simulink model "double_pend"  (R2019b)
settings: Solver=VariableStepAuto  StartTime=0.0  StopTime=10.0  RelTol=1e-3
values from neighbouring files (symbols this model uses):
  Bd = 50    [anujay_single_pendulum_same.m]    (also in connect_pend_runner.m; double_pend_setup.m = [50,0;0,50])
  dampener = 100    [anujay_single_pendulum_same.m]    (also in connect_pend.m; connect_pend_runner.m; double_pend_setup.m = [50, 0; 0, 50])
  Dm1 = 30    [anujay_single_pendulum_same.m]    (also in connect_pend.m; connect_pend_runner.m; double_pend_setup.m = [30,0;0,30])
  Kd = 50    [anujay_single_pendulum_same.m]    (also in connect_pend_runner.m; double_pend_setup.m = [50,0;0,50]; single_pend_runner.m = 500)
  Ked = 50    [anujay_single_pendulum_same.m]    (also in double_pend_setup.m = [ 100, 0; 0, 100])
  Kem = 50    [anujay_single_pendulum_same.m]    (also in double_pend_setup.m = [100, 0; 0, 100])
  Km1 = 30    [anujay_single_pendulum_same.m]    (also in connect_pend.m; connect_pend_runner.m; double_pend_setup.m = [30, 0; 0 30])
  l = [ 1.0, 1.5]    [double_pend_setup.m]
  l1 = 1.0    (= 1)    [connect_pend.m]    (also in connect_pend_runner.m; run.m)
  l2 = l1    (= 1)    [connect_pend_runner.m]    (also in single_pend_runner.m = 3)
  lambda2 = 1.2    [anujay_single_pendulum_same.m]    (also in connect_pend_runner.m = 3; double_pend_setup.m = [1.5, 0; 0 1.5])
  Md = 10    [anujay_single_pendulum_same.m]    (also in connect_pend_runner.m; double_pend_setup.m = [10, 0; 0, 10])
  me = 2.11  + mh    (= 13.934)    [anujay_single_pendulum_same.m]    (also in double_pend_setup.m = [ 2, 1] + mh)
  mh = 11.824    [anujay_single_pendulum_same.m]    (also in double_pend_setup.m = [2, 1])
  rho2 = 100    [anujay_single_pendulum_same.m]    (also in connect_pend_runner.m = 15; double_pend_setup.m = [100, 0; 0, 100])
  sat = 10    [double_pend_setup.m]
  spring = 100    [anujay_single_pendulum_same.m]    (also in connect_pend.m; connect_pend_runner.m; double_pend_setup.m = [50, 0; 0, 50])
undefined symbols (not defined in the file or in its folder): me2
libraries: simulink x2, robotcorelib x1
settings Model: Creator=nathanielgoldfarb  LastModifiedBy=nathanielgoldfarb
settings SolverCC: ZeroCrossAlgorithm=Adaptive
settings DebuggingCC: IgnoredZcDiagnostic=none  UnderSpecifiedDimensionMsg=warning

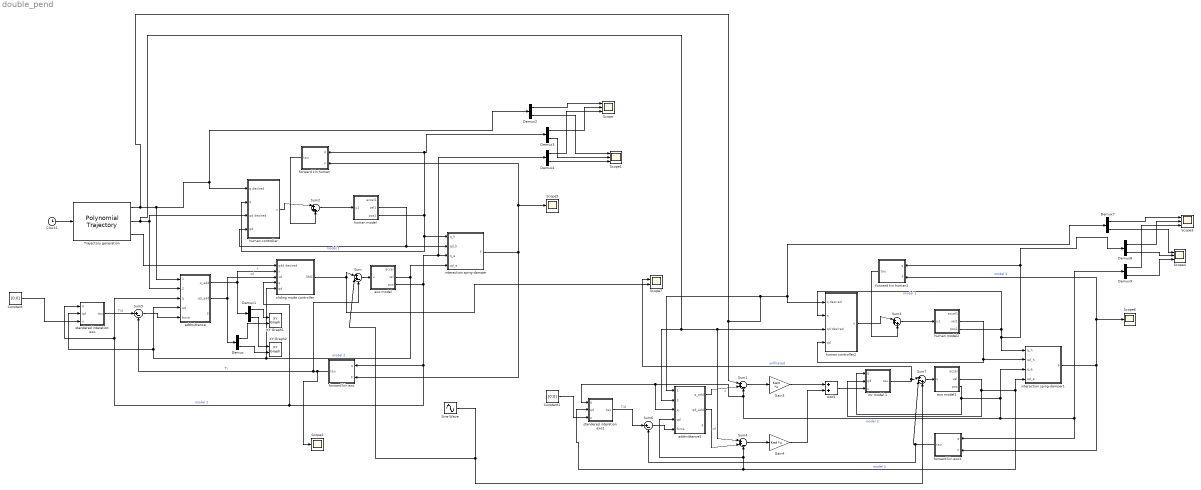
== system double_pend ==
  " interaction sping-damper" : Subsystem
  " interaction sping-damper1" : Subsystem
  Add1 : Sum
  Clock1 : Clock
  Constant : Constant  Value=[0;0]
  Constant1 : Constant  Value=[0;0]
  Demux{,1..4,7..9} (8 alike) : Demux  Outputs=2
  Gain3 : Gain  Gain=Kem  Multiplication=Matrix(K*u)
  Gain4 : Gain  Gain=Ked  Multiplication=Matrix(K*u)
  Scope{,1,3..4} (4 alike) : Scope  NumInputPorts=3
  Scope2 : Scope
  Scope5 : Scope
  Scope6 : Scope
  Scope7 : Scope  NumInputPorts=2
  Sine Wave : Sin  Amplitude=0  Frequency=4  SampleTime=0
  Sum : Sum  Inputs=|++-
  Sum1 : Sum  Inputs=|++-
  Sum2 : Sum  Inputs=|+++
  Sum3 : Sum  Inputs=|+++
  Sum4 : Sum  Inputs=|++-
  Sum5 : Sum  Inputs=|+-
  Sum6 : Sum  Inputs=|+-
  Sum7 : Sum  Inputs=|+-+
  Trajectory generation : robotcorelib/Polynomial Trajectory  WaypointSource=Internal  Waypoints="[ 0 , -pi;  0 -0.5*pi ]"  TimePoints=[ 0, 3]  TimeInterval=[ 1, 4 ]  Method=Cubic Polynomial  ParameterSource=Internal  VelocityBoundaryCondition=zeros( 2, 2 )  AccelerationBoundaryCondition=zeros( 2, 5 )  SimulateUsing=Interpreted execution
      settings: SourceProductName=Robotics System Toolbox  SourceProductBaseCode=RO
  XY Graph1 : simulink/Sinks/XY Graph  xmin=-5  xmax=5  ymin=-3  ymax=3  st=-1
  XY Graph2 : simulink/Sinks/XY Graph  xmin=-3  xmax=0.5  ymin=-2  ymax=2.2  st=-1
  addmittance : Subsystem
  addmittance1 : Subsystem
  exo model : Subsystem
  exo model1 : Subsystem
  forward kin exo : Subsystem
  forward kin exo1 : Subsystem
  forward kin human : Subsystem
  forward kin human1 : Subsystem
  human controller : Subsystem
  human controller2 : Subsystem
  human model : Subsystem
  human model2 : Subsystem
  inv model 1 : Subsystem
  sliding mode controller : Subsystem
  standered interation exo : Subsystem
  standered interation exo1 : Subsystem
  wires:
  addmittance/1(q_add) -> Demux1/1, sliding mode controller/2(x)  "x"
  Clock1/1 -> Trajectory generation/1
  Trajectory generation/3 -> sliding mode controller/1(qdd desired)
  human model/3(pos1) -> human controller/2(q), " interaction sping-damper"/1(q_h), Demux3/1, forward kin human/1(q)  "model 1"
  human model/2(vel1) -> human controller/4(qd), " interaction sping-damper"/2(qd_h)
  forward kin human/1(tau) -> Sum2/3
  " interaction sping-damper"/1(F) -> forward kin exo/2(F), forward kin human/2(F), Scope5/1
  exo model/2(vel) -> " interaction sping-damper"/4("qd_e "), standered interation exo/2(qd), addmittance/4(qd), sliding mode controller/5(qd)  "model 2"
  Sum5/1 -> addmittance/5(force)
  exo model/3(pos) -> Demux4/1, " interaction sping-damper"/3(q_e), sliding mode controller/4(q), standered interation exo/1(q), addmittance/3(q), forward kin exo/1(q)  "model 2"
  addmittance/2(qd_add) -> Demux/1, sliding mode controller/3(xd)  "xd"
  standered interation exo/1("tau ") -> Sum5/1  "Tid"
  Constant/1 -> standered interation exo/3("u ")
  Demux/2 -> XY Graph2/2
  Demux/1 -> XY Graph1/2
  Demux1/1 -> XY Graph1/1
  Demux1/2 -> XY Graph2/1
  forward kin exo/1(tau) -> Scope2/1, Sum5/2, Sum/3  "Ti"
  Demux2/1 -> Scope/1
  Demux3/1 -> Scope/2
  Demux4/1 -> Scope/3
  Demux2/2 -> Scope1/1
  Demux3/2 -> Scope1/2
  Demux4/2 -> Scope1/3
  exo model1/2(vel) -> inv model 1/2(qd), " interaction sping-damper1"/4("qd_e "), Sum4/3, addmittance1/4(qd), standered interation exo1/2(qd)  "model 2"
  Demux7/2 -> Scope4/1
  Demux9/1 -> Scope3/3
  forward kin human1/1(tau) -> Sum3/3
  Demux7/1 -> Scope3/1
  Demux8/2 -> Scope4/2
  exo model1/3(pos) -> inv model 1/1(q), " interaction sping-damper1"/3(q_e), Sum1/3, addmittance1/3(q), standered interation exo1/1(q), Demux9/1, forward kin exo1/1(q)  "model 2"
  Demux9/2 -> Scope4/3
  human model2/3(pos1) -> " interaction sping-damper1"/1(q_h), forward kin human1/1(q), Demux8/1, human controller2/2(q)  "model 1"
  Demux8/1 -> Scope3/2
  human model2/2(vel1) -> human controller2/4(qd), " interaction sping-damper1"/2(qd_h)
  Trajectory generation/1 -> Demux7/1, human controller2/1(q desired), addmittance1/1(q desird), Sum1/1, addmittance/1(q desird), human controller/1(q desired), Demux2/1
  " interaction sping-damper1"/1(F) -> forward kin exo1/2(F), forward kin human1/2(F), Scope6/1  "model 2"
  Sum4/1 -> Gain4/1
  Gain4/1 -> Add1/2
  Trajectory generation/2 -> addmittance1/2(qd desird), Sum4/1, human controller2/3(qd desired), human controller/3(qd desired), addmittance/2(qd desird)
  Gain3/1 -> Add1/1
  Sum1/1 -> Gain3/1
  Sine Wave/1 -> Sum7/3, Sum/2
  human controller/1(u) -> Sum2/1
  Sum2/1 -> human model/1(u1)
  human controller2/1(u) -> Sum3/1
  Sum3/1 -> human model2/1(u1)
  Add1/1 -> inv model 1/3("u ")
  inv model 1/1("tau ") -> Sum7/1, Scope7/1  "unfiltered"
  Sum7/1 -> exo model1/1(u)
  forward kin exo1/1(tau) -> Sum6/2, Sum7/2
  Sum/1 -> exo model/1(u)
  sliding mode controller/1(SMC) -> Sum/1, Scope7/2
  Constant1/1 -> standered interation exo1/3("u ")
  standered interation exo1/1("tau ") -> Sum6/1  "Tid"
  addmittance1/1(q_add) -> Sum1/2  "x"
  addmittance1/2(qd_add) -> Sum4/2  "xd"
  Sum6/1 -> addmittance1/5(force)

== system double_pend/ interaction sping-damper ==
  q_h : Inport
  qd_h : Inport  Port=2
  q_e : Inport  Port=3
  "qd_e " : Inport  Port=4
  Mux : Mux  Inputs=2
  Subsystem : Subsystem
  Subsystem1 : Subsystem
  forward kin : Subsystem
  forward kin2 : Subsystem
  F : Outport
  wires:
  qd_h/1 -> forward kin/2(qd)
  q_h/1 -> forward kin/1("q ")
  "qd_e "/1 -> forward kin2/2(qd)
  q_e/1 -> forward kin2/1("q ")
  forward kin/1(pos1) -> Subsystem/1(x human)
  forward kin/3(vel1) -> Subsystem/2("xd human ")
  forward kin2/1(pos1) -> Subsystem/3(x exo)
  forward kin2/3(vel1) -> Subsystem/4(xd exo)
  forward kin/2(pos2) -> Subsystem1/1(x human)
  forward kin2/2(pos2) -> Subsystem1/3(x exo)
  forward kin/4(vel2) -> Subsystem1/2("xd human ")
  forward kin2/4(vel2) -> Subsystem1/4(xd exo)
  Subsystem/1(F) -> Mux/1
  Subsystem1/1(F) -> Mux/2
  Mux/1 -> F/1

== system double_pend/ interaction sping-damper1 ==
  q_h : Inport
  qd_h : Inport  Port=2
  q_e : Inport  Port=3
  "qd_e " : Inport  Port=4
  Mux : Mux  Inputs=2
  Subsystem : Subsystem
  Subsystem1 : Subsystem
  forward kin : Subsystem
  forward kin2 : Subsystem
  F : Outport
  wires:
  qd_h/1 -> forward kin/2(qd)
  q_h/1 -> forward kin/1("q ")
  "qd_e "/1 -> forward kin2/2(qd)
  q_e/1 -> forward kin2/1("q ")
  forward kin/1(pos1) -> Subsystem/1(x human)
  forward kin/3(vel1) -> Subsystem/2("xd human ")
  forward kin2/1(pos1) -> Subsystem/3(x exo)
  forward kin2/3(vel1) -> Subsystem/4(xd exo)
  forward kin/2(pos2) -> Subsystem1/1(x human)
  forward kin2/2(pos2) -> Subsystem1/3(x exo)
  forward kin/4(vel2) -> Subsystem1/2("xd human ")
  forward kin2/4(vel2) -> Subsystem1/4(xd exo)
  Subsystem/1(F) -> Mux/1
  Subsystem1/1(F) -> Mux/2
  Mux/1 -> F/1

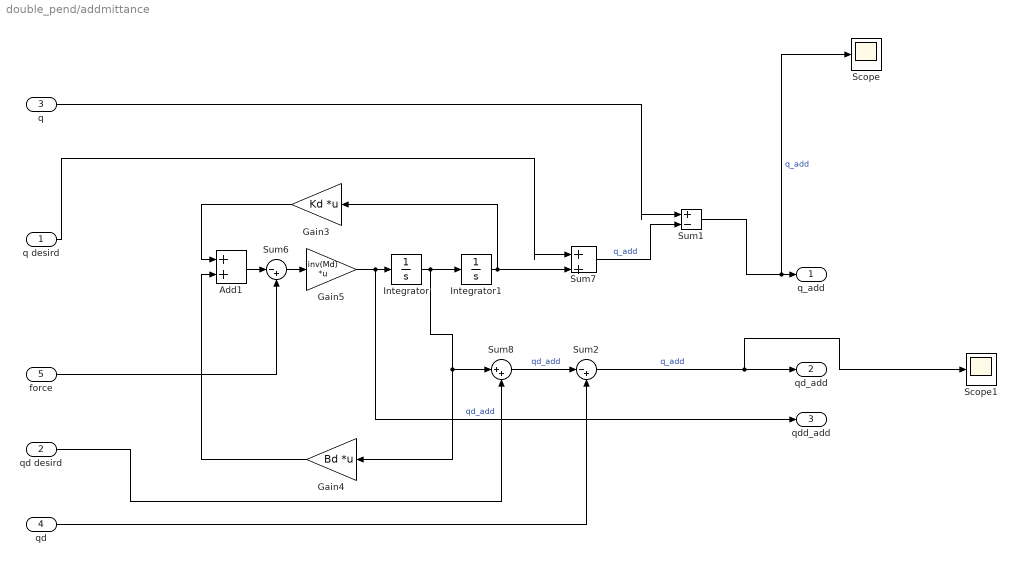
== system double_pend/addmittance ==
  q desird : Inport
  qd desird : Inport  Port=2
  q : Inport  Port=3
  qd : Inport  Port=4
  force : Inport  Port=5
  Add1 : Sum
  Gain3 : Gain  Gain=Kd  Multiplication=Matrix(K*u)
  Gain4 : Gain  Gain=Bd  Multiplication=Matrix(K*u)
  Gain5 : Gain  Gain=inv(Md)  Multiplication=Matrix(K*u)
  Integrator : Integrator
  Integrator1 : Integrator  InitialCondition=[-pi, 0.5*pi]
  Scope : Scope
  Scope1 : Scope
  Sum1 : Sum  Inputs=|+-
  Sum2 : Sum  Inputs=|-+
  Sum6 : Sum  Inputs=|-+
  Sum7 : Sum  Inputs=|++
  Sum8 : Sum  Inputs=|++
  q_add : Outport
  qd_add : Outport  Port=2
  qdd_add : Outport  Port=3
  wires:
  Add1/1 -> Sum6/1
  force/1 -> Sum6/2
  qd desird/1 -> Sum8/2
  Gain5/1 -> qdd_add/1, Integrator/1  "qd_add"
  Sum6/1 -> Gain5/1
  Gain4/1 -> Add1/2
  Gain3/1 -> Add1/1
  Integrator/1 -> Gain4/1, Sum8/1, Integrator1/1
  q desird/1 -> Sum7/1
  Integrator1/1 -> Sum7/2, Gain3/1
  qd/1 -> Sum2/2
  Sum2/1 -> Scope1/1, qd_add/1  "q_add"
  Sum7/1 -> Sum1/2  "q_add"
  q/1 -> Sum1/1
  Sum1/1 -> Scope/1, q_add/1  "q_add"
  Sum8/1 -> Sum2/1  "qd_add"

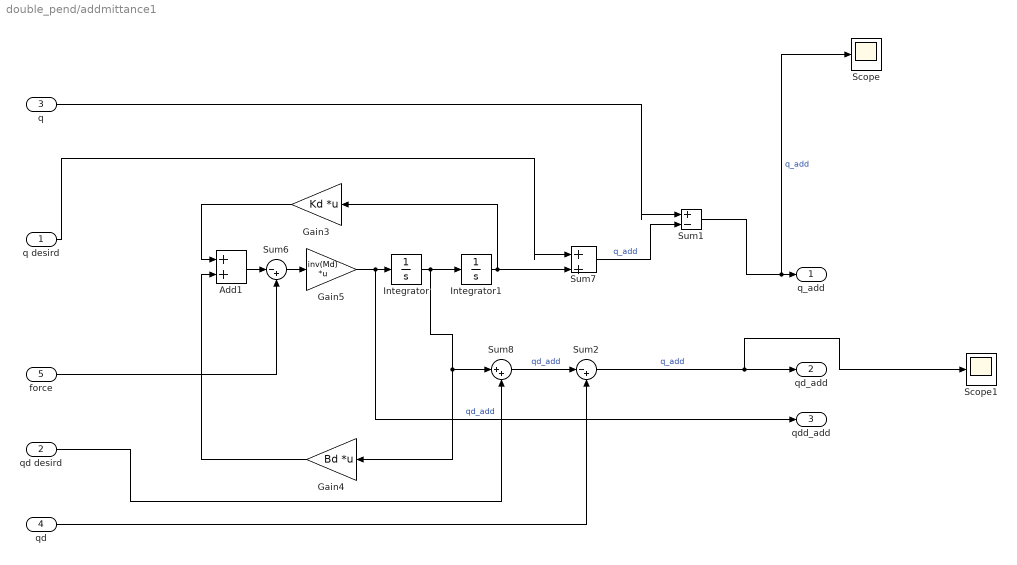
== system double_pend/addmittance1 ==
  q desird : Inport
  qd desird : Inport  Port=2
  q : Inport  Port=3
  qd : Inport  Port=4
  force : Inport  Port=5
  Add1 : Sum
  Gain3 : Gain  Gain=Kd  Multiplication=Matrix(K*u)
  Gain4 : Gain  Gain=Bd  Multiplication=Matrix(K*u)
  Gain5 : Gain  Gain=inv(Md)  Multiplication=Matrix(K*u)
  Integrator : Integrator
  Integrator1 : Integrator  InitialCondition=[-pi, 0.5*pi]
  Scope : Scope
  Scope1 : Scope
  Sum1 : Sum  Inputs=|+-
  Sum2 : Sum  Inputs=|-+
  Sum6 : Sum  Inputs=|-+
  Sum7 : Sum  Inputs=|++
  Sum8 : Sum  Inputs=|++
  q_add : Outport
  qd_add : Outport  Port=2
  qdd_add : Outport  Port=3
  wires:
  Add1/1 -> Sum6/1
  force/1 -> Sum6/2
  qd desird/1 -> Sum8/2
  Gain5/1 -> qdd_add/1, Integrator/1  "qd_add"
  Sum6/1 -> Gain5/1
  Gain4/1 -> Add1/2
  Gain3/1 -> Add1/1
  Integrator/1 -> Gain4/1, Sum8/1, Integrator1/1
  q desird/1 -> Sum7/1
  Integrator1/1 -> Sum7/2, Gain3/1
  qd/1 -> Sum2/2
  Sum2/1 -> Scope1/1, qd_add/1  "q_add"
  Sum7/1 -> Sum1/2  "q_add"
  q/1 -> Sum1/1
  Sum1/1 -> Scope/1, q_add/1  "q_add"
  Sum8/1 -> Sum2/1  "qd_add"

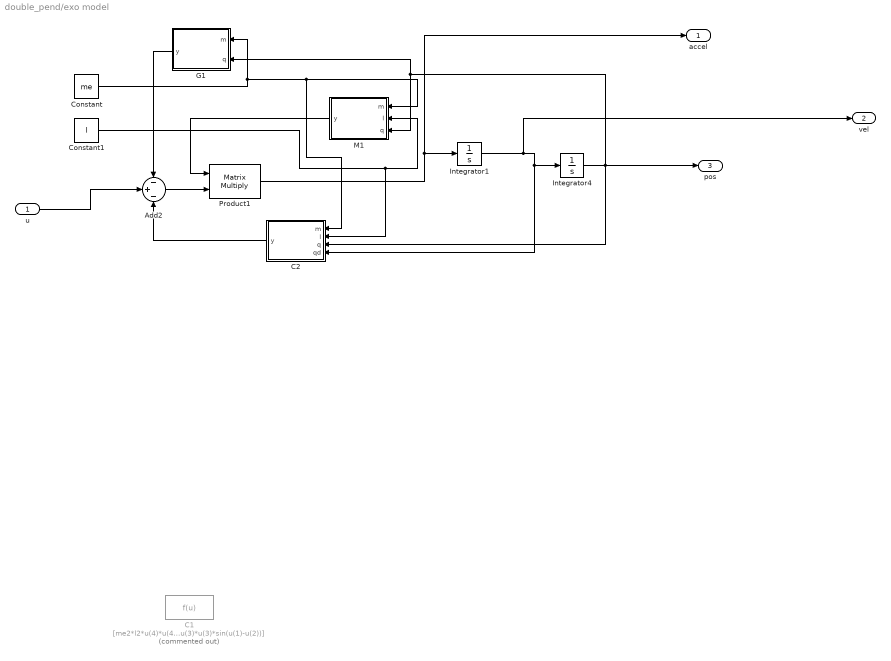
== system double_pend/exo model ==
  u : Inport
  Add2 : Sum  Inputs=-+-
  C1 : Fcn  Commented=on  Expr=[me2*l2*u(4)*u(4)*sin(u(1)-u(2)); -me2*l1*u(3)*u(3)*sin(u(1)-u(2))]
  C2 : MATLAB Function  TreatAsAtomicUnit=on
  Constant : Constant  Value=me
  Constant1 : Constant  Value=l
  G1 : MATLAB Function  TreatAsAtomicUnit=on
  Integrator1 : Integrator  InitialCondition=[0;0]
  Integrator4 : Integrator  InitialCondition=[0.01;0.01]
  M1 : MATLAB Function  TreatAsAtomicUnit=on
  Product1 : Product  Multiplication=Matrix(*)
  accel : Outport
  vel : Outport  Port=2
  pos : Outport  Port=3
  wires:
  Constant/1 -> C2/1(m), M1/1(m), G1/1(m)
  M1/1(y) -> Product1/1
  Add2/1 -> Product1/2
  C2/1(y) -> Add2/3
  G1/1(y) -> Add2/1
  u/1 -> Add2/2
  Product1/1 -> accel/1, Integrator1/1
  Constant1/1 -> C2/2(l), M1/2(l)
  Integrator4/1 -> pos/1, G1/2(q), M1/3(q), C2/3(q)
  Integrator1/1 -> vel/1, C2/4(qd), Integrator4/1

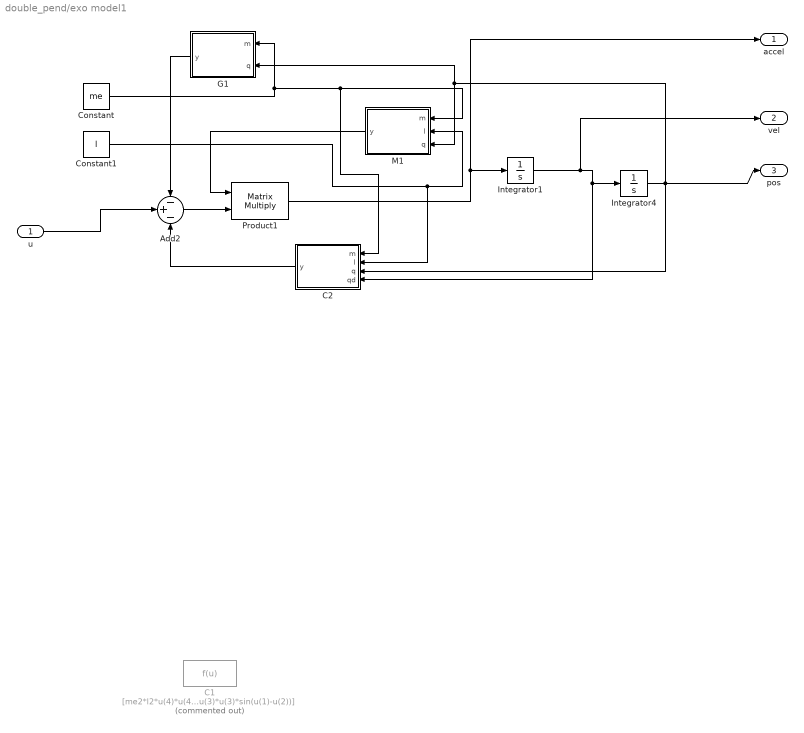
== system double_pend/exo model1 ==
  u : Inport
  Add2 : Sum  Inputs=-+-
  C1 : Fcn  Commented=on  Expr=[me2*l2*u(4)*u(4)*sin(u(1)-u(2)); -me2*l1*u(3)*u(3)*sin(u(1)-u(2))]
  C2 : MATLAB Function  TreatAsAtomicUnit=on
  Constant : Constant  Value=me
  Constant1 : Constant  Value=l
  G1 : MATLAB Function  TreatAsAtomicUnit=on
  Integrator1 : Integrator  InitialCondition=[0;0]
  Integrator4 : Integrator  InitialCondition=[0.01;0.01]
  M1 : MATLAB Function  TreatAsAtomicUnit=on
  Product1 : Product  Multiplication=Matrix(*)
  accel : Outport
  vel : Outport  Port=2
  pos : Outport  Port=3
  wires:
  Constant/1 -> C2/1(m), M1/1(m), G1/1(m)
  M1/1(y) -> Product1/1
  Add2/1 -> Product1/2
  C2/1(y) -> Add2/3
  G1/1(y) -> Add2/1
  u/1 -> Add2/2
  Product1/1 -> accel/1, Integrator1/1
  Constant1/1 -> C2/2(l), M1/2(l)
  Integrator1/1 -> vel/1, C2/4(qd), Integrator4/1
  Integrator4/1 -> pos/1, G1/2(q), M1/3(q), C2/3(q)

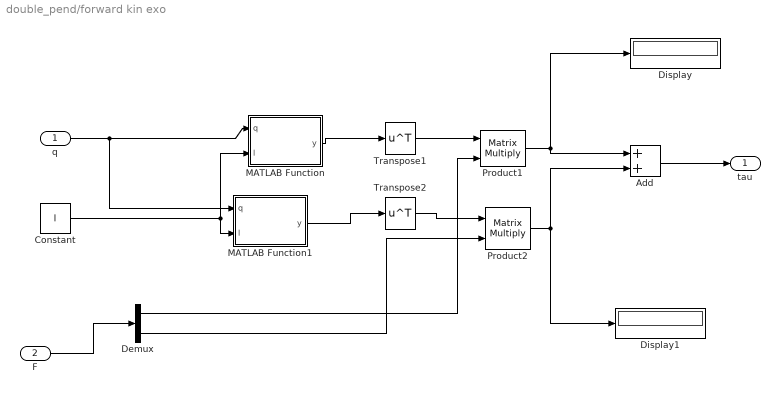
== system double_pend/forward kin exo ==
  q : Inport
  F : Inport  Port=2
  Add : Sum
  Constant : Constant  Value=l
  Demux : Demux  Outputs=2
  Display : Display
  Display1 : Display
  MATLAB Function : MATLAB Function  TreatAsAtomicUnit=on
  MATLAB Function1 : MATLAB Function  TreatAsAtomicUnit=on
  Product1 : Product  Multiplication=Matrix(*)
  Product2 : Product  Multiplication=Matrix(*)
  Transpose1 : Math  Operator=transpose  SignedPower=off  SaturateOnIntegerOverflow=on
  Transpose2 : Math  Operator=transpose  SignedPower=off  SaturateOnIntegerOverflow=on
  tau : Outport
  wires:
  Product1/1 -> Add/1, Display/1
  F/1 -> Demux/1
  q/1 -> MATLAB Function1/1(q), MATLAB Function/1(q)
  Constant/1 -> MATLAB Function/2(l), MATLAB Function1/2(l)
  Add/1 -> tau/1
  Demux/2 -> Product2/2
  Transpose2/1 -> Product2/1
  Demux/1 -> Product1/2
  Product2/1 -> Add/2, Display1/1
  MATLAB Function1/1(y) -> Transpose2/1
  MATLAB Function/1(y) -> Transpose1/1
  Transpose1/1 -> Product1/1

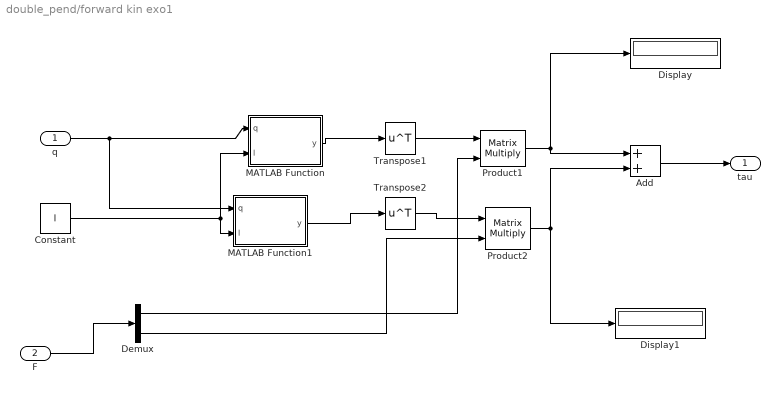
== system double_pend/forward kin exo1 ==
  q : Inport
  F : Inport  Port=2
  Add : Sum
  Constant : Constant  Value=l
  Demux : Demux  Outputs=2
  Display : Display
  Display1 : Display
  MATLAB Function : MATLAB Function  TreatAsAtomicUnit=on
  MATLAB Function1 : MATLAB Function  TreatAsAtomicUnit=on
  Product1 : Product  Multiplication=Matrix(*)
  Product2 : Product  Multiplication=Matrix(*)
  Transpose1 : Math  Operator=transpose  SignedPower=off  SaturateOnIntegerOverflow=on
  Transpose2 : Math  Operator=transpose  SignedPower=off  SaturateOnIntegerOverflow=on
  tau : Outport
  wires:
  Product1/1 -> Add/1, Display/1
  F/1 -> Demux/1
  q/1 -> MATLAB Function1/1(q), MATLAB Function/1(q)
  Constant/1 -> MATLAB Function/2(l), MATLAB Function1/2(l)
  Add/1 -> tau/1
  Demux/2 -> Product2/2
  Transpose2/1 -> Product2/1
  Demux/1 -> Product1/2
  Product2/1 -> Add/2, Display1/1
  MATLAB Function1/1(y) -> Transpose2/1
  MATLAB Function/1(y) -> Transpose1/1
  Transpose1/1 -> Product1/1

== system double_pend/forward kin human ==
  q : Inport
  F : Inport  Port=2
  Add : Sum
  Constant : Constant  Value=l
  Demux : Demux  Outputs=2
  Display : Display
  Display1 : Display
  MATLAB Function : MATLAB Function  TreatAsAtomicUnit=on
  MATLAB Function1 : MATLAB Function  TreatAsAtomicUnit=on
  Product1 : Product  Multiplication=Matrix(*)
  Product2 : Product  Multiplication=Matrix(*)
  Transpose1 : Math  Operator=transpose  SignedPower=off  SaturateOnIntegerOverflow=on
  Transpose2 : Math  Operator=transpose  SignedPower=off  SaturateOnIntegerOverflow=on
  tau : Outport
  wires:
  q/1 -> MATLAB Function1/1(q), MATLAB Function/1(q)
  Demux/2 -> Product2/2
  F/1 -> Demux/1
  Demux/1 -> Product1/2
  Transpose1/1 -> Product1/1
  Transpose2/1 -> Product2/1
  MATLAB Function1/1(y) -> Transpose2/1
  MATLAB Function/1(y) -> Transpose1/1
  Constant/1 -> MATLAB Function/2(l), MATLAB Function1/2(l)
  Add/1 -> tau/1
  Product1/1 -> Add/1, Display/1
  Product2/1 -> Add/2, Display1/1

== system double_pend/forward kin human1 ==
  q : Inport
  F : Inport  Port=2
  Add : Sum
  Constant : Constant  Value=l
  Demux : Demux  Outputs=2
  Display : Display
  Display1 : Display
  MATLAB Function : MATLAB Function  TreatAsAtomicUnit=on
  MATLAB Function1 : MATLAB Function  TreatAsAtomicUnit=on
  Product1 : Product  Multiplication=Matrix(*)
  Product2 : Product  Multiplication=Matrix(*)
  Transpose1 : Math  Operator=transpose  SignedPower=off  SaturateOnIntegerOverflow=on
  Transpose2 : Math  Operator=transpose  SignedPower=off  SaturateOnIntegerOverflow=on
  tau : Outport
  wires:
  q/1 -> MATLAB Function1/1(q), MATLAB Function/1(q)
  Demux/2 -> Product2/2
  F/1 -> Demux/1
  Demux/1 -> Product1/2
  Transpose1/1 -> Product1/1
  Transpose2/1 -> Product2/1
  MATLAB Function1/1(y) -> Transpose2/1
  MATLAB Function/1(y) -> Transpose1/1
  Constant/1 -> MATLAB Function/2(l), MATLAB Function1/2(l)
  Add/1 -> tau/1
  Product1/1 -> Add/1, Display/1
  Product2/1 -> Add/2, Display1/1

== system double_pend/human controller ==
  q desired : Inport
  q : Inport  Port=2
  qd desired : Inport  Port=3
  qd : Inport  Port=4
  Add2 : Sum
  Gain1 : Gain  Gain=Km1  Multiplication=Matrix(K*u)
  Gain2 : Gain  Gain=Dm1  Multiplication=Matrix(K*u)
  Saturation : Saturate  UpperLimit=sat  LowerLimit=-sat
  Scope2 : Scope  NumInputPorts=3
  Sum1 : Sum  Inputs=|+-
  Sum3 : Sum  Inputs=|-+
  inv model 1 : Subsystem
  u : Outport
  wires:
  Sum1/1 -> Gain2/1
  qd/1 -> inv model 1/2(qd), Sum1/2
  Sum3/1 -> Gain1/1
  Gain2/1 -> Add2/2
  q desired/1 -> Sum3/2
  Add2/1 -> inv model 1/3("u ")
  Gain1/1 -> Add2/1
  inv model 1/1("tau ") -> Scope2/1, Saturation/1  "unfiltered"
  qd desired/1 -> Sum1/1
  q/1 -> Sum3/1, inv model 1/1(q)
  Saturation/1 -> u/1, Scope2/3, Scope2/2  "filtered"

== system double_pend/human controller2 ==
  q desired : Inport
  q : Inport  Port=2
  qd desired : Inport  Port=3
  qd : Inport  Port=4
  Add2 : Sum
  Gain1 : Gain  Gain=Km1  Multiplication=Matrix(K*u)
  Gain2 : Gain  Gain=Dm1  Multiplication=Matrix(K*u)
  Saturation : Saturate  UpperLimit=sat  LowerLimit=-sat
  Scope2 : Scope  NumInputPorts=3
  Sum1 : Sum  Inputs=|+-
  Sum3 : Sum  Inputs=|-+
  inv model 1 : Subsystem
  u : Outport
  wires:
  Sum1/1 -> Gain2/1
  qd/1 -> inv model 1/2(qd), Sum1/2
  Sum3/1 -> Gain1/1
  Gain2/1 -> Add2/2
  q desired/1 -> Sum3/2
  Add2/1 -> inv model 1/3("u ")
  Gain1/1 -> Add2/1
  inv model 1/1("tau ") -> Scope2/1, Saturation/1  "unfiltered"
  qd desired/1 -> Sum1/1
  q/1 -> Sum3/1, inv model 1/1(q)
  Saturation/1 -> u/1, Scope2/3, Scope2/2  "filtered"

== system double_pend/human model ==
  u1 : Inport
  Add2 : Sum  Inputs=-+-
  C : MATLAB Function  TreatAsAtomicUnit=on
  Constant : Constant  Value=mh
  Constant1 : Constant  Value=l
  G : MATLAB Function  TreatAsAtomicUnit=on
  Integrator1 : Integrator  InitialCondition=[0;0]
  Integrator4 : Integrator  InitialCondition=[0.01;0.01]
  M : MATLAB Function  TreatAsAtomicUnit=on
  Product1 : Product  Multiplication=Matrix(*)
  accel1 : Outport
  vel1 : Outport  Port=2
  pos1 : Outport  Port=3
  wires:
  C/1(y) -> Add2/3
  M/1(y) -> Product1/1
  G/1(y) -> Add2/1
  Integrator4/1 -> C/3(q), pos1/1, G/2(q), M/3(q)
  u1/1 -> Add2/2
  Product1/1 -> accel1/1, Integrator1/1
  Integrator1/1 -> vel1/1, C/4(qd), Integrator4/1
  Add2/1 -> Product1/2
  Constant/1 -> C/1(m), M/1(m), G/1(m)
  Constant1/1 -> C/2(l), M/2(l)

== system double_pend/human model2 ==
  u1 : Inport
  Add2 : Sum  Inputs=-+-
  C : MATLAB Function  TreatAsAtomicUnit=on
  Constant : Constant  Value=mh
  Constant1 : Constant  Value=l
  G : MATLAB Function  TreatAsAtomicUnit=on
  Integrator1 : Integrator  InitialCondition=[0;0]
  Integrator4 : Integrator  InitialCondition=[0.01;0.01]
  M : MATLAB Function  TreatAsAtomicUnit=on
  Product1 : Product  Multiplication=Matrix(*)
  accel1 : Outport
  vel1 : Outport  Port=2
  pos1 : Outport  Port=3
  wires:
  C/1(y) -> Add2/3
  M/1(y) -> Product1/1
  G/1(y) -> Add2/1
  Integrator4/1 -> C/3(q), pos1/1, G/2(q), M/3(q)
  u1/1 -> Add2/2
  Product1/1 -> accel1/1, Integrator1/1
  Integrator1/1 -> vel1/1, C/4(qd), Integrator4/1
  Add2/1 -> Product1/2
  Constant/1 -> C/1(m), M/1(m), G/1(m)
  Constant1/1 -> C/2(l), M/2(l)

== system double_pend/inv model 1 ==
  q : Inport
  qd : Inport  Port=2
  "u " : Inport  Port=3
  Add2 : Sum  Inputs=+++
  C2 : MATLAB Function  TreatAsAtomicUnit=on
  Constant : Constant  Value=me
  Constant1 : Constant  Value=l
  G1 : MATLAB Function  TreatAsAtomicUnit=on
  M1 : MATLAB Function  TreatAsAtomicUnit=on
  Product : Product  Multiplication=Matrix(*)
  "tau " : Outport
  wires:
  G1/1(y) -> Add2/3
  C2/1(y) -> Add2/2
  q/1 -> G1/2(q), C2/3(q), M1/3(q)
  qd/1 -> C2/4(qd)
  M1/1(y) -> Product/1
  Product/1 -> Add2/1
  Constant/1 -> G1/1(m), C2/1(m), M1/1(m)
  Constant1/1 -> C2/2(l), M1/2(l)
  "u "/1 -> Product/2
  Add2/1 -> "tau "/1

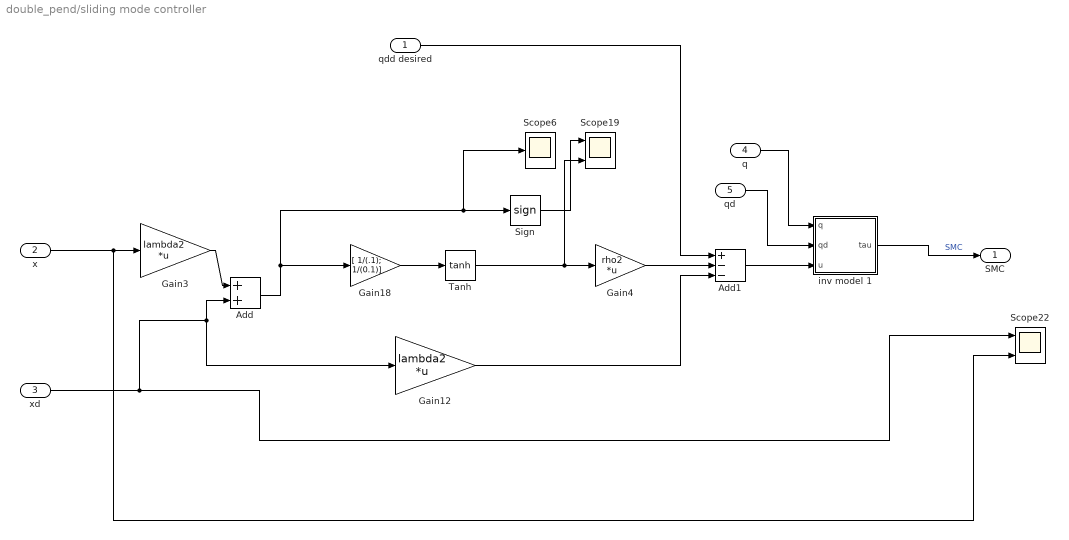
== system double_pend/sliding mode controller ==
  qdd desired : Inport
  x : Inport  Port=2
  xd : Inport  Port=3
  q : Inport  Port=4
  qd : Inport  Port=5
  Add : Sum
  Add1 : Sum  Inputs=+--
  Gain12 : Gain  Gain=lambda2  Multiplication=Matrix(K*u)
  Gain18 : Gain  Gain=[ 1/(.1); 1/(0.1)]
  Gain3 : Gain  Gain=lambda2  Multiplication=Matrix(K*u)
  Gain4 : Gain  Gain=rho2  Multiplication=Matrix(K*u)
  Scope19 : Scope  NumInputPorts=2
  Scope22 : Scope  NumInputPorts=2
  Scope6 : Scope
  Sign : Signum
  Tanh : Trigonometry  Operator=tanh
  inv model 1 : Subsystem
  SMC : Outport
  wires:
  Gain18/1 -> Tanh/1
  Gain12/1 -> Add1/3
  Gain3/1 -> Add/1
  inv model 1/1("tau ") -> SMC/1  "SMC"
  x/1 -> Scope22/2, Gain3/1
  xd/1 -> Add/2, Gain12/1, Scope22/1
  Add/1 -> Scope6/1, Sign/1, Gain18/1
  Add1/1 -> inv model 1/3("u ")
  Sign/1 -> Scope19/1
  Gain4/1 -> Add1/2
  qdd desired/1 -> Add1/1
  Tanh/1 -> Gain4/1, Scope19/2
  q/1 -> inv model 1/1(q)
  qd/1 -> inv model 1/2(qd)

== system double_pend/standered interation exo ==
  q : Inport
  qd : Inport  Port=2
  "u " : Inport  Port=3
  Add2 : Sum  Inputs=+++
  C2 : MATLAB Function  TreatAsAtomicUnit=on
  Constant : Constant  Value=me
  Constant1 : Constant  Value=l
  G1 : MATLAB Function  TreatAsAtomicUnit=on
  M : MATLAB Function  TreatAsAtomicUnit=on
  Product : Product  Multiplication=Matrix(*)
  "tau " : Outport
  wires:
  Add2/1 -> "tau "/1
  C2/1(y) -> Add2/2
  Product/1 -> Add2/1
  G1/1(y) -> Add2/3
  q/1 -> G1/2(q), C2/3(q), M/3(q)
  Constant/1 -> C2/1(m), M/1(m), G1/1(m)
  M/1(y) -> Product/1
  "u "/1 -> Product/2
  qd/1 -> C2/4(qd)
  Constant1/1 -> C2/2(l), M/2(l)

== system double_pend/standered interation exo1 ==
  q : Inport
  qd : Inport  Port=2
  "u " : Inport  Port=3
  Add2 : Sum  Inputs=+++
  C2 : MATLAB Function  TreatAsAtomicUnit=on
  Constant : Constant  Value=me
  Constant1 : Constant  Value=l
  G1 : MATLAB Function  TreatAsAtomicUnit=on
  M : MATLAB Function  TreatAsAtomicUnit=on
  Product : Product  Multiplication=Matrix(*)
  "tau " : Outport
  wires:
  Add2/1 -> "tau "/1
  C2/1(y) -> Add2/2
  Product/1 -> Add2/1
  G1/1(y) -> Add2/3
  q/1 -> G1/2(q), C2/3(q), M/3(q)
  Constant/1 -> C2/1(m), M/1(m), G1/1(m)
  M/1(y) -> Product/1
  "u "/1 -> Product/2
  qd/1 -> C2/4(qd)
  Constant1/1 -> C2/2(l), M/2(l)

== system double_pend/ interaction sping-damper/Subsystem ==
  x human : Inport
  "xd human " : Inport  Port=2
  x exo : Inport  Port=3
  xd exo : Inport  Port=4
  Gain3 : Gain  Gain=spring  Multiplication=Matrix(K*u)
  Gain4 : Gain  Gain=dampener  Multiplication=Matrix(K*u)
  Subtract : Sum  Inputs=-+
  Subtract1 : Sum  Inputs=-+
  Subtract2 : Sum
  F : Outport
  wires:
  Subtract2/1 -> F/1
  xd exo/1 -> Subtract1/2
  Gain4/1 -> Subtract2/2
  Subtract/1 -> Gain3/1
  Subtract1/1 -> Gain4/1
  x exo/1 -> Subtract/2
  x human/1 -> Subtract/1
  "xd human "/1 -> Subtract1/1
  Gain3/1 -> Subtract2/1

== system double_pend/ interaction sping-damper/Subsystem1 ==
  x human : Inport
  "xd human " : Inport  Port=2
  x exo : Inport  Port=3
  xd exo : Inport  Port=4
  Gain3 : Gain  Gain=spring  Multiplication=Matrix(K*u)
  Gain4 : Gain  Gain=dampener  Multiplication=Matrix(K*u)
  Subtract : Sum  Inputs=-+
  Subtract1 : Sum  Inputs=-+
  Subtract2 : Sum
  F : Outport
  wires:
  Subtract2/1 -> F/1
  xd exo/1 -> Subtract1/2
  Gain4/1 -> Subtract2/2
  Subtract/1 -> Gain3/1
  Subtract1/1 -> Gain4/1
  x exo/1 -> Subtract/2
  x human/1 -> Subtract/1
  "xd human "/1 -> Subtract1/1
  Gain3/1 -> Subtract2/1

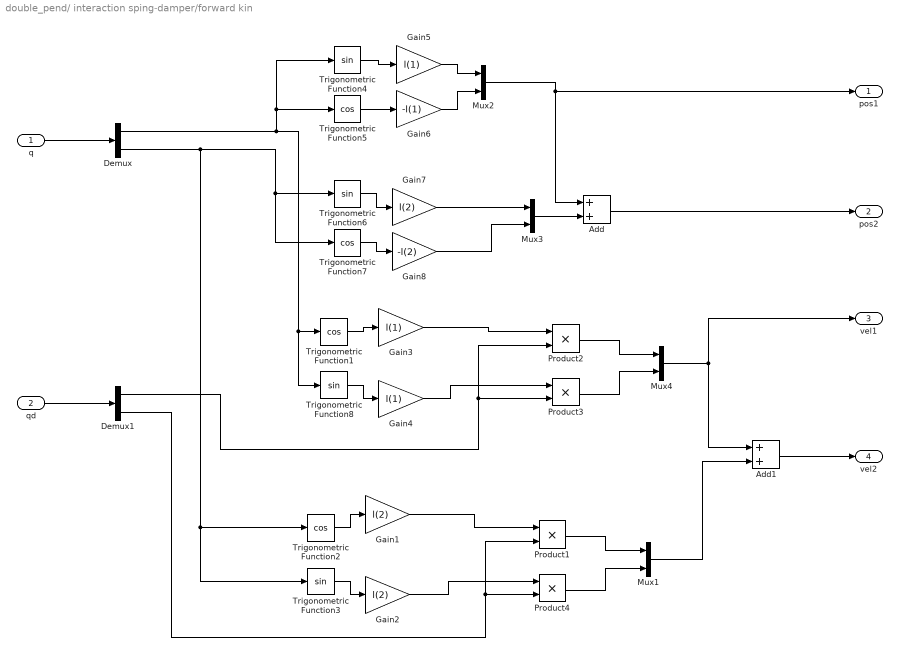
== system double_pend/ interaction sping-damper/forward kin ==
  "q " : Inport
  qd : Inport  Port=2
  Add : Sum
  Add1 : Sum
  Demux : Demux  Outputs=2
  Demux1 : Demux  Outputs=2
  Gain1 : Gain  Gain=l(2)
  Gain2 : Gain  Gain=l(2)
  Gain3 : Gain  Gain=l(1)
  Gain4 : Gain  Gain=l(1)
  Gain5 : Gain  Gain=l(1)
  Gain6 : Gain  Gain=-l(1)
  Gain7 : Gain  Gain=l(2)
  Gain8 : Gain  Gain=-l(2)
  Mux{1..4} (4 alike) : Mux  Inputs=2
  Product{1..4} (4 alike) : Product
  Trigonometric Function{1..2,5,7} (4 alike) : Trigonometry  Operator=cos
  Trigonometric Function{3..4,6,8} (4 alike) : Trigonometry
  pos1 : Outport
  pos2 : Outport  Port=2
  vel1 : Outport  Port=3
  vel2 : Outport  Port=4
  wires:
  "q "/1 -> Demux/1
  qd/1 -> Demux1/1
  Gain6/1 -> Mux2/2
  Trigonometric Function4/1 -> Gain5/1
  Gain5/1 -> Mux2/1
  Trigonometric Function5/1 -> Gain6/1
  Demux/1 -> Trigonometric Function8/1, Trigonometric Function1/1, Trigonometric Function5/1, Trigonometric Function4/1
  Trigonometric Function6/1 -> Gain7/1
  Gain8/1 -> Mux3/2
  Trigonometric Function7/1 -> Gain8/1
  Demux/2 -> Trigonometric Function3/1, Trigonometric Function2/1, Trigonometric Function7/1, Trigonometric Function6/1
  Gain7/1 -> Mux3/1
  Mux3/1 -> Add/2
  Trigonometric Function1/1 -> Gain3/1
  Gain3/1 -> Product2/1
  Demux1/1 -> Product3/2, Product2/2
  Trigonometric Function8/1 -> Gain4/1
  Gain4/1 -> Product3/1
  Product2/1 -> Mux4/1
  Product3/1 -> Mux4/2
  Trigonometric Function3/1 -> Gain2/1
  Trigonometric Function2/1 -> Gain1/1
  Product4/1 -> Mux1/2
  Demux1/2 -> Product4/2, Product1/2
  Gain2/1 -> Product4/1
  Product1/1 -> Mux1/1
  Gain1/1 -> Product1/1
  Mux4/1 -> Add1/1, vel1/1
  Mux1/1 -> Add1/2
  Add/1 -> pos2/1
  Mux2/1 -> Add/1, pos1/1
  Add1/1 -> vel2/1

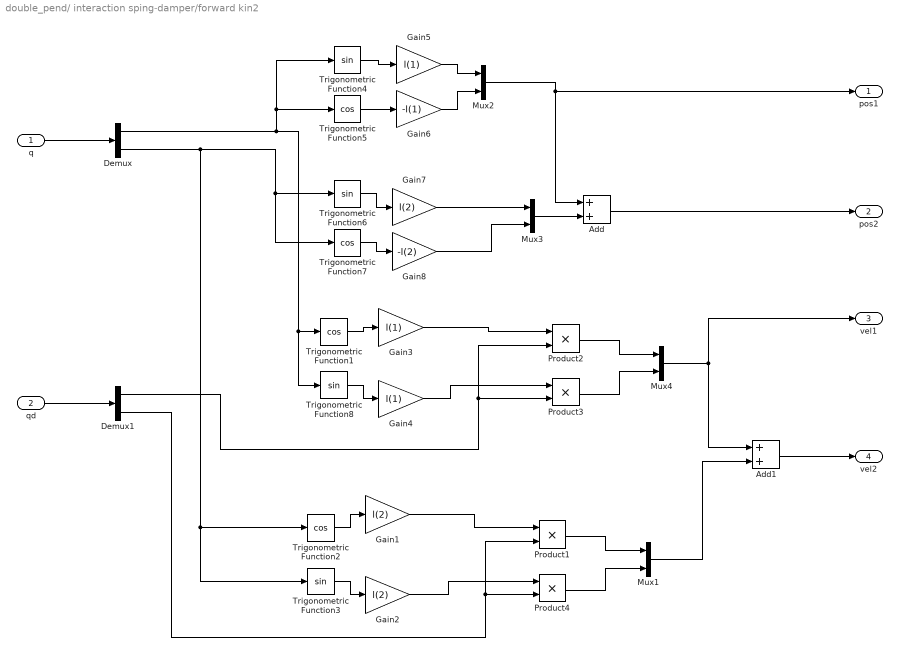
== system double_pend/ interaction sping-damper/forward kin2 ==
  "q " : Inport
  qd : Inport  Port=2
  Add : Sum
  Add1 : Sum
  Demux : Demux  Outputs=2
  Demux1 : Demux  Outputs=2
  Gain1 : Gain  Gain=l(2)
  Gain2 : Gain  Gain=l(2)
  Gain3 : Gain  Gain=l(1)
  Gain4 : Gain  Gain=l(1)
  Gain5 : Gain  Gain=l(1)
  Gain6 : Gain  Gain=-l(1)
  Gain7 : Gain  Gain=l(2)
  Gain8 : Gain  Gain=-l(2)
  Mux{1..4} (4 alike) : Mux  Inputs=2
  Product{1..4} (4 alike) : Product
  Trigonometric Function{1..2,5,7} (4 alike) : Trigonometry  Operator=cos
  Trigonometric Function{3..4,6,8} (4 alike) : Trigonometry
  pos1 : Outport
  pos2 : Outport  Port=2
  vel1 : Outport  Port=3
  vel2 : Outport  Port=4
  wires:
  "q "/1 -> Demux/1
  qd/1 -> Demux1/1
  Gain6/1 -> Mux2/2
  Trigonometric Function4/1 -> Gain5/1
  Gain5/1 -> Mux2/1
  Trigonometric Function5/1 -> Gain6/1
  Demux/1 -> Trigonometric Function8/1, Trigonometric Function1/1, Trigonometric Function5/1, Trigonometric Function4/1
  Trigonometric Function6/1 -> Gain7/1
  Gain8/1 -> Mux3/2
  Trigonometric Function7/1 -> Gain8/1
  Demux/2 -> Trigonometric Function3/1, Trigonometric Function2/1, Trigonometric Function7/1, Trigonometric Function6/1
  Gain7/1 -> Mux3/1
  Mux3/1 -> Add/2
  Trigonometric Function1/1 -> Gain3/1
  Gain3/1 -> Product2/1
  Demux1/1 -> Product3/2, Product2/2
  Trigonometric Function8/1 -> Gain4/1
  Gain4/1 -> Product3/1
  Product2/1 -> Mux4/1
  Product3/1 -> Mux4/2
  Trigonometric Function3/1 -> Gain2/1
  Trigonometric Function2/1 -> Gain1/1
  Product4/1 -> Mux1/2
  Demux1/2 -> Product4/2, Product1/2
  Gain2/1 -> Product4/1
  Product1/1 -> Mux1/1
  Gain1/1 -> Product1/1
  Mux4/1 -> Add1/1, vel1/1
  Mux1/1 -> Add1/2
  Add/1 -> pos2/1
  Mux2/1 -> Add/1, pos1/1
  Add1/1 -> vel2/1

== system double_pend/ interaction sping-damper1/Subsystem ==
  x human : Inport
  "xd human " : Inport  Port=2
  x exo : Inport  Port=3
  xd exo : Inport  Port=4
  Gain3 : Gain  Gain=spring  Multiplication=Matrix(K*u)
  Gain4 : Gain  Gain=dampener  Multiplication=Matrix(K*u)
  Subtract : Sum  Inputs=-+
  Subtract1 : Sum  Inputs=-+
  Subtract2 : Sum
  F : Outport
  wires:
  Subtract2/1 -> F/1
  xd exo/1 -> Subtract1/2
  Gain4/1 -> Subtract2/2
  Subtract/1 -> Gain3/1
  Subtract1/1 -> Gain4/1
  x exo/1 -> Subtract/2
  x human/1 -> Subtract/1
  "xd human "/1 -> Subtract1/1
  Gain3/1 -> Subtract2/1

== system double_pend/ interaction sping-damper1/Subsystem1 ==
  x human : Inport
  "xd human " : Inport  Port=2
  x exo : Inport  Port=3
  xd exo : Inport  Port=4
  Gain3 : Gain  Gain=spring  Multiplication=Matrix(K*u)
  Gain4 : Gain  Gain=dampener  Multiplication=Matrix(K*u)
  Subtract : Sum  Inputs=-+
  Subtract1 : Sum  Inputs=-+
  Subtract2 : Sum
  F : Outport
  wires:
  Subtract2/1 -> F/1
  xd exo/1 -> Subtract1/2
  Gain4/1 -> Subtract2/2
  Subtract/1 -> Gain3/1
  Subtract1/1 -> Gain4/1
  x exo/1 -> Subtract/2
  x human/1 -> Subtract/1
  "xd human "/1 -> Subtract1/1
  Gain3/1 -> Subtract2/1

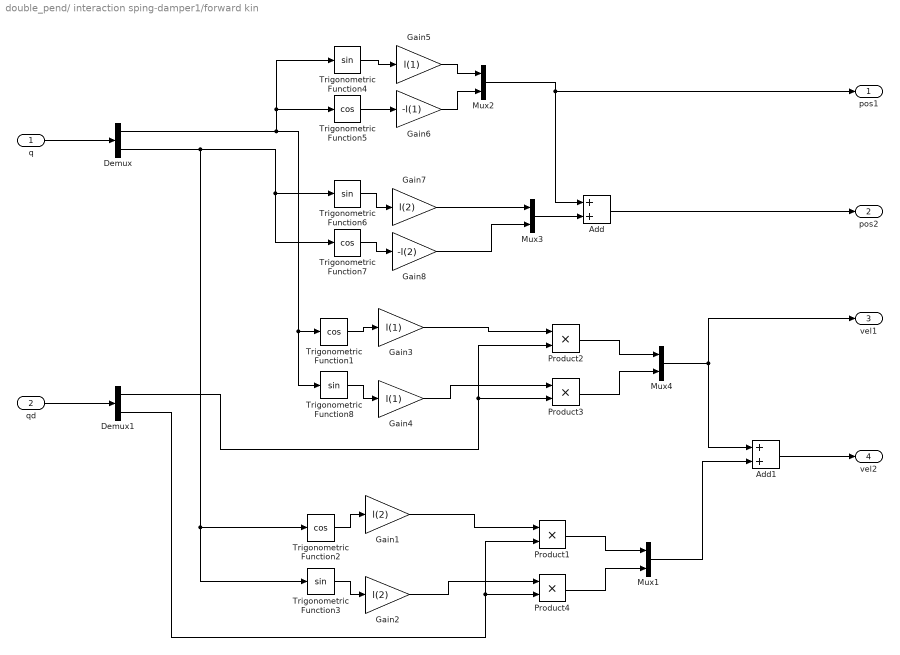
== system double_pend/ interaction sping-damper1/forward kin ==
  "q " : Inport
  qd : Inport  Port=2
  Add : Sum
  Add1 : Sum
  Demux : Demux  Outputs=2
  Demux1 : Demux  Outputs=2
  Gain1 : Gain  Gain=l(2)
  Gain2 : Gain  Gain=l(2)
  Gain3 : Gain  Gain=l(1)
  Gain4 : Gain  Gain=l(1)
  Gain5 : Gain  Gain=l(1)
  Gain6 : Gain  Gain=-l(1)
  Gain7 : Gain  Gain=l(2)
  Gain8 : Gain  Gain=-l(2)
  Mux{1..4} (4 alike) : Mux  Inputs=2
  Product{1..4} (4 alike) : Product
  Trigonometric Function{1..2,5,7} (4 alike) : Trigonometry  Operator=cos
  Trigonometric Function{3..4,6,8} (4 alike) : Trigonometry
  pos1 : Outport
  pos2 : Outport  Port=2
  vel1 : Outport  Port=3
  vel2 : Outport  Port=4
  wires:
  "q "/1 -> Demux/1
  qd/1 -> Demux1/1
  Gain6/1 -> Mux2/2
  Trigonometric Function4/1 -> Gain5/1
  Gain5/1 -> Mux2/1
  Trigonometric Function5/1 -> Gain6/1
  Demux/1 -> Trigonometric Function8/1, Trigonometric Function1/1, Trigonometric Function5/1, Trigonometric Function4/1
  Trigonometric Function6/1 -> Gain7/1
  Gain8/1 -> Mux3/2
  Trigonometric Function7/1 -> Gain8/1
  Demux/2 -> Trigonometric Function3/1, Trigonometric Function2/1, Trigonometric Function7/1, Trigonometric Function6/1
  Gain7/1 -> Mux3/1
  Mux3/1 -> Add/2
  Trigonometric Function1/1 -> Gain3/1
  Gain3/1 -> Product2/1
  Demux1/1 -> Product3/2, Product2/2
  Trigonometric Function8/1 -> Gain4/1
  Gain4/1 -> Product3/1
  Product2/1 -> Mux4/1
  Product3/1 -> Mux4/2
  Trigonometric Function3/1 -> Gain2/1
  Trigonometric Function2/1 -> Gain1/1
  Product4/1 -> Mux1/2
  Demux1/2 -> Product4/2, Product1/2
  Gain2/1 -> Product4/1
  Product1/1 -> Mux1/1
  Gain1/1 -> Product1/1
  Mux4/1 -> Add1/1, vel1/1
  Mux1/1 -> Add1/2
  Add/1 -> pos2/1
  Mux2/1 -> Add/1, pos1/1
  Add1/1 -> vel2/1

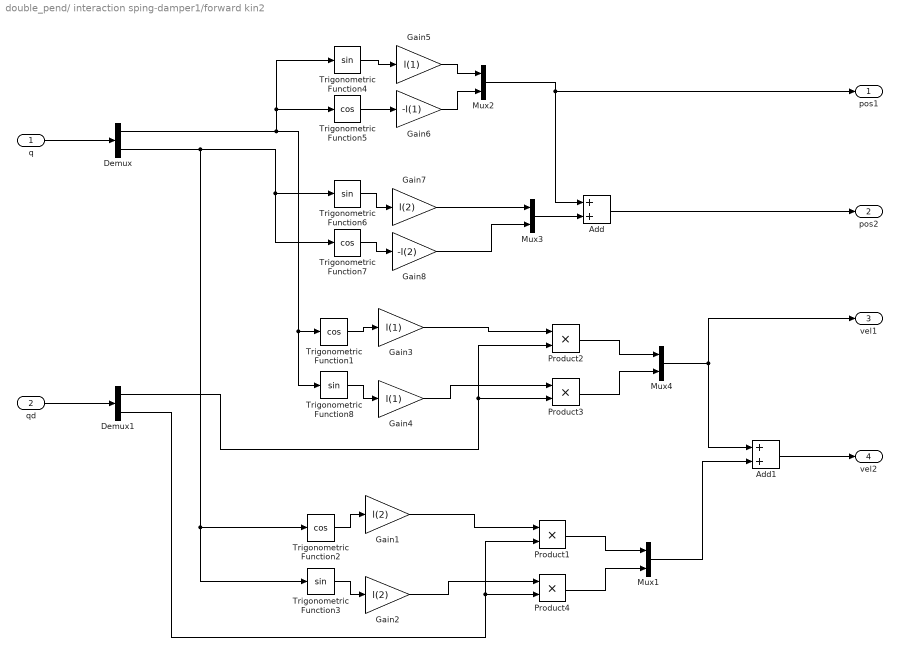
== system double_pend/ interaction sping-damper1/forward kin2 ==
  "q " : Inport
  qd : Inport  Port=2
  Add : Sum
  Add1 : Sum
  Demux : Demux  Outputs=2
  Demux1 : Demux  Outputs=2
  Gain1 : Gain  Gain=l(2)
  Gain2 : Gain  Gain=l(2)
  Gain3 : Gain  Gain=l(1)
  Gain4 : Gain  Gain=l(1)
  Gain5 : Gain  Gain=l(1)
  Gain6 : Gain  Gain=-l(1)
  Gain7 : Gain  Gain=l(2)
  Gain8 : Gain  Gain=-l(2)
  Mux{1..4} (4 alike) : Mux  Inputs=2
  Product{1..4} (4 alike) : Product
  Trigonometric Function{1..2,5,7} (4 alike) : Trigonometry  Operator=cos
  Trigonometric Function{3..4,6,8} (4 alike) : Trigonometry
  pos1 : Outport
  pos2 : Outport  Port=2
  vel1 : Outport  Port=3
  vel2 : Outport  Port=4
  wires:
  "q "/1 -> Demux/1
  qd/1 -> Demux1/1
  Gain6/1 -> Mux2/2
  Trigonometric Function4/1 -> Gain5/1
  Gain5/1 -> Mux2/1
  Trigonometric Function5/1 -> Gain6/1
  Demux/1 -> Trigonometric Function8/1, Trigonometric Function1/1, Trigonometric Function5/1, Trigonometric Function4/1
  Trigonometric Function6/1 -> Gain7/1
  Gain8/1 -> Mux3/2
  Trigonometric Function7/1 -> Gain8/1
  Demux/2 -> Trigonometric Function3/1, Trigonometric Function2/1, Trigonometric Function7/1, Trigonometric Function6/1
  Gain7/1 -> Mux3/1
  Mux3/1 -> Add/2
  Trigonometric Function1/1 -> Gain3/1
  Gain3/1 -> Product2/1
  Demux1/1 -> Product3/2, Product2/2
  Trigonometric Function8/1 -> Gain4/1
  Gain4/1 -> Product3/1
  Product2/1 -> Mux4/1
  Product3/1 -> Mux4/2
  Trigonometric Function3/1 -> Gain2/1
  Trigonometric Function2/1 -> Gain1/1
  Product4/1 -> Mux1/2
  Demux1/2 -> Product4/2, Product1/2
  Gain2/1 -> Product4/1
  Product1/1 -> Mux1/1
  Gain1/1 -> Product1/1
  Mux4/1 -> Add1/1, vel1/1
  Mux1/1 -> Add1/2
  Add/1 -> pos2/1
  Mux2/1 -> Add/1, pos1/1
  Add1/1 -> vel2/1

== system double_pend/human controller/inv model 1 ==
  q : Inport
  qd : Inport  Port=2
  "u " : Inport  Port=3
  Add2 : Sum  Inputs=+++
  C2 : MATLAB Function  TreatAsAtomicUnit=on
  Constant : Constant  Value=mh
  Constant1 : Constant  Value=l
  G1 : MATLAB Function  TreatAsAtomicUnit=on
  M1 : MATLAB Function  TreatAsAtomicUnit=on
  Product : Product  Multiplication=Matrix(*)
  "tau " : Outport
  wires:
  G1/1(y) -> Add2/3
  C2/1(y) -> Add2/2
  Add2/1 -> "tau "/1
  q/1 -> G1/2(q), C2/3(q), M1/3(q)
  qd/1 -> C2/4(qd)
  M1/1(y) -> Product/1
  Product/1 -> Add2/1
  "u "/1 -> Product/2
  Constant/1 -> G1/1(m), C2/1(m), M1/1(m)
  Constant1/1 -> C2/2(l), M1/2(l)

== system double_pend/human controller2/inv model 1 ==
  q : Inport
  qd : Inport  Port=2
  "u " : Inport  Port=3
  Add2 : Sum  Inputs=+++
  C2 : MATLAB Function  TreatAsAtomicUnit=on
  Constant : Constant  Value=mh
  Constant1 : Constant  Value=l
  G1 : MATLAB Function  TreatAsAtomicUnit=on
  M1 : MATLAB Function  TreatAsAtomicUnit=on
  Product : Product  Multiplication=Matrix(*)
  "tau " : Outport
  wires:
  G1/1(y) -> Add2/3
  C2/1(y) -> Add2/2
  Add2/1 -> "tau "/1
  q/1 -> G1/2(q), C2/3(q), M1/3(q)
  qd/1 -> C2/4(qd)
  M1/1(y) -> Product/1
  Product/1 -> Add2/1
  "u "/1 -> Product/2
  Constant/1 -> G1/1(m), C2/1(m), M1/1(m)
  Constant1/1 -> C2/2(l), M1/2(l)

== system double_pend/sliding mode controller/inv model 1 ==
  q : Inport
  qd : Inport  Port=2
  "u " : Inport  Port=3
  Add2 : Sum  Inputs=+++
  C2 : MATLAB Function  TreatAsAtomicUnit=on
  Constant : Constant  Value=me
  Constant1 : Constant  Value=l
  G1 : MATLAB Function  TreatAsAtomicUnit=on
  M1 : MATLAB Function  TreatAsAtomicUnit=on
  Product : Product  Multiplication=Matrix(*)
  "tau " : Outport
  wires:
  G1/1(y) -> Add2/3
  C2/1(y) -> Add2/2
  Add2/1 -> "tau "/1
  q/1 -> G1/2(q), C2/3(q), M1/3(q)
  qd/1 -> C2/4(qd)
  M1/1(y) -> Product/1
  Product/1 -> Add2/1
  "u "/1 -> Product/2
  Constant/1 -> G1/1(m), C2/1(m), M1/1(m)
  Constant1/1 -> C2/2(l), M1/2(l)

== matlab function double_pend/human controller/inv model 1/C2 ==
  data: m input; l input; q input; y output; qd input
function y = fcn(m, l, q, qd)

y = [m(2)*l(2)*qd(2)*qd(2)*sin(q(1)-q(2)); -m(2)*l(1)*qd(1)*qd(1)*sin(q(1)-q(2))];

== matlab function double_pend/human controller/inv model 1/G1 ==
  data: m input; q input; y output
function y = fcn(m, q)

g = -9.81;

y =[ (m(1)+m(2))*g*sin(q(1)); m(2)*g*sin(q(1))] ;

== matlab function double_pend/human controller/inv model 1/M1 ==
  data: m input; l input; q input; y output
function y = fcn(m, l, q)


y =[ (m(1)+m(2)) *l(1), m(2)*cos(q(1)-q(2)); m(2)*l(1)*cos(q(1)-q(2)), m(2)*l(2)] ;

== matlab function double_pend/human model/C ==
  data: m input; l input; q input; y output; qd input
function y = fcn(m, l, q, qd)



y = [m(2)*l(2)*qd(2)*qd(2)*sin(q(1)-q(2)); -m(2)*l(1)*qd(1)*qd(1)*sin(q(1)-q(2))];

== matlab function double_pend/human model/G ==
  data: m input; q input; y output
function y = fcn(m, q)
g = -9.81;                  % Needed in order to set variable class correctly

y =[ (m(1)+m(2))*g*sin(q(1)); m(2)*g*sin(q(1))] ;

== matlab function double_pend/human model/M ==
  data: m input; l input; q input; y output
function y = fcn(m, l, q)

y = pinv([ (m(1)+m(2)) *l(1), m(2)*cos(q(1)-q(2)); m(2)*l(1)*cos(q(1)-q(2)), m(2)*l(2)] );

== matlab function double_pend/forward kin exo/MATLAB Function ==
  data: q input; y output; l input
function y = fcn(q,l)

y = [l(1)*cos(q(1)), 0; l(1)*sin(q(1)), 0 ];

== matlab function double_pend/standered interation exo/C2 ==
  data: m input; l input; q input; y output; qd input
function y = fcn(m, l, q, qd)



y = [m(2)*l(2)*qd(2)*qd(2)*sin(q(1)-q(2)); -m(2)*l(1)*qd(1)*qd(1)*sin(q(1)-q(2))];

== matlab function double_pend/standered interation exo/G1 ==
  data: m input; q input; y output
function y = fcn(m, q)

g = -9.81;

y =[ (m(1)+m(2))*g*sin(q(1)); m(2)*g*sin(q(1))] ;

== matlab function double_pend/standered interation exo/M ==
  data: m input; l input; q input; y output
function y = fcn(m, l, q)

y =[ (m(1)+m(2)) *l(1), m(2)*cos(q(1)-q(2)); m(2)*l(1)*cos(q(1)-q(2)), m(2)*l(2)] ;

== matlab function double_pend/forward kin exo/MATLAB Function1 ==
  data: q input; y output; l input
function y = fcn(q, l)


y = [l(1)*cos(q(1)), l(2)*cos(q(2)) ; l(1)*sin(q(1)), l(2)*sin(q(2)) ];

== matlab function double_pend/forward kin human/MATLAB Function ==
  data: q input; y output; l input
function y = fcn(q,l)

y = [l(1)*cos(q(1)), 0; l(1)*sin(q(1)), 0 ];

== matlab function double_pend/forward kin human/MATLAB Function1 ==
  data: q input; y output; l input
function y = fcn(q, l)


y = [l(1)*cos(q(1)), l(2)*cos(q(2)) ; l(1)*sin(q(1)), l(2)*sin(q(2)) ];

== matlab function double_pend/sliding mode controller/inv model 1/C2 ==
  data: m input; l input; q input; y output; qd input
function y = fcn(m, l, q, qd)

y =  [m(2)*l(2)*qd(2)*qd(2)*sin(q(1)-q(2)); -m(2)*l(1)*qd(1)*qd(1)*sin(q(1)-q(2))];

== matlab function double_pend/sliding mode controller/inv model 1/G1 ==
  data: m input; q input; y output
function y = fcn(m, q)

g = -9.81;

y = [ (m(1)+m(2))*g*sin(q(1)); m(2)*g*sin(q(1))] ;

== matlab function double_pend/sliding mode controller/inv model 1/M1 ==
  data: m input; l input; q input; y output
function y = fcn(m, l, q)


y =   [ (m(1)+m(2)) *l(1), m(2)*cos(q(1)-q(2)); m(2)*l(1)*cos(q(1)-q(2)), m(2)*l(2)] ;

== matlab function double_pend/exo model/C2 ==
  data: m input; l input; q input; y output; qd input
function y = fcn(m, l, q, qd)


y = [m(2)*l(2)*qd(2)*qd(2)*sin(q(1)-q(2)); -m(2)*l(1)*qd(1)*qd(1)*sin(q(1)-q(2))];

== matlab function double_pend/exo model/G1 ==
  data: m input; q input; y output
function y = fcn(m, q)
g = -9.81;


y =[ (m(1)+m(2))*g*sin(q(1)); m(2)*g*sin(q(1))] ;

== matlab function double_pend/exo model/M1 ==
  data: m input; l input; q input; y output
function y = fcn(m, l, q)


y = pinv([ (m(1)+m(2)) *l(1), m(2)*cos(q(1)-q(2)); m(2)*l(1)*cos(q(1)-q(2)), m(2)*l(2)] );

== matlab function double_pend/exo model1/C2 ==
  data: m input; l input; q input; y output; qd input
function y = fcn(m, l, q, qd)


y = [m(2)*l(2)*qd(2)*qd(2)*sin(q(1)-q(2)); -m(2)*l(1)*qd(1)*qd(1)*sin(q(1)-q(2))];

== matlab function double_pend/exo model1/G1 ==
  data: m input; q input; y output
function y = fcn(m, q)
g = -9.81;


y =[ (m(1)+m(2))*g*sin(q(1)); m(2)*g*sin(q(1))] ;

== matlab function double_pend/exo model1/M1 ==
  data: m input; l input; q input; y output
function y = fcn(m, l, q)



y = pinv( [ (m(1)+m(2)) *l(1), m(2)*cos(q(1)-q(2)); m(2)*l(1)*cos(q(1)-q(2)), m(2)*l(2)] );

== matlab function double_pend/forward kin exo1/MATLAB Function ==
  data: q input; y output; l input
function y = fcn(q,l)

y = [l(1)*cos(q(1)), 0; l(1)*sin(q(1)), 0 ];

== matlab function double_pend/standered interation exo1/C2 ==
  data: m input; l input; q input; y output; qd input
function y = fcn(m, l, q, qd)



y = [m(2)*l(2)*qd(2)*qd(2)*sin(q(1)-q(2)); -m(2)*l(1)*qd(1)*qd(1)*sin(q(1)-q(2))];

== matlab function double_pend/standered interation exo1/G1 ==
  data: m input; q input; y output
function y = fcn(m, q)

g = -9.81;

y =[ (m(1)+m(2))*g*sin(q(1)); m(2)*g*sin(q(1))] ;

== matlab function double_pend/standered interation exo1/M ==
  data: m input; l input; q input; y output
function y = fcn(m, l, q)

y =[ (m(1)+m(2)) *l(1), m(2)*cos(q(1)-q(2)); m(2)*l(1)*cos(q(1)-q(2)), m(2)*l(2)] ;

== matlab function double_pend/forward kin exo1/MATLAB Function1 ==
  data: q input; y output; l input
function y = fcn(q, l)


y = [l(1)*cos(q(1)), l(2)*cos(q(2)) ; l(1)*sin(q(1)), l(2)*sin(q(2)) ];

== matlab function double_pend/forward kin human1/MATLAB Function ==
  data: q input; y output; l input
function y = fcn(q,l)

y = [l(1)*cos(q(1)), 0; l(1)*sin(q(1)), 0 ];

== matlab function double_pend/forward kin human1/MATLAB Function1 ==
  data: q input; y output; l input
function y = fcn(q, l)


y = [l(1)*cos(q(1)), l(2)*cos(q(2)) ; l(1)*sin(q(1)), l(2)*sin(q(2)) ];

== matlab function double_pend/human controller2/inv model 1/C2 ==
  data: m input; l input; q input; y output; qd input
function y = fcn(m, l, q, qd)

y = [m(2)*l(2)*qd(2)*qd(2)*sin(q(1)-q(2)); -m(2)*l(1)*qd(1)*qd(1)*sin(q(1)-q(2))];

== matlab function double_pend/human controller2/inv model 1/G1 ==
  data: m input; q input; y output
function y = fcn(m, q)

g = -9.81;

y =[ (m(1)+m(2))*g*sin(q(1)); m(2)*g*sin(q(1))] ;

== matlab function double_pend/human controller2/inv model 1/M1 ==
  data: m input; l input; q input; y output
function y = fcn(m, l, q)


y =[ (m(1)+m(2)) *l(1), m(2)*cos(q(1)-q(2)); m(2)*l(1)*cos(q(1)-q(2)), m(2)*l(2)] ;

== matlab function double_pend/human model2/C ==
  data: m input; l input; q input; y output; qd input
function y = fcn(m, l, q, qd)



y = [m(2)*l(2)*qd(2)*qd(2)*sin(q(1)-q(2)); -m(2)*l(1)*qd(1)*qd(1)*sin(q(1)-q(2))];

== matlab function double_pend/human model2/G ==
  data: m input; q input; y output
function y = fcn(m, q)
g = -9.81;                  % Needed in order to set variable class correctly

y =[ (m(1)+m(2))*g*sin(q(1)); m(2)*g*sin(q(1))] ;

== matlab function double_pend/human model2/M ==
  data: m input; l input; q input; y output
function y = fcn(m, l, q)

y = pinv([ (m(1)+m(2)) *l(1), m(2)*cos(q(1)-q(2)); m(2)*l(1)*cos(q(1)-q(2)), m(2)*l(2)] );

== matlab function double_pend/inv model 1/C2 ==
  data: m input; l input; q input; y output; qd input
function y = fcn(m, l, q, qd)

y = [m(2)*l(2)*qd(2)*qd(2)*sin(q(1)-q(2)); -m(2)*l(1)*qd(1)*qd(1)*sin(q(1)-q(2))];

== matlab function double_pend/inv model 1/G1 ==
  data: m input; q input; y output
function y = fcn(m, q)

g = -9.81;

y =  [ (m(1)+m(2))*g*sin(q(1)); m(2)*g*sin(q(1))] ;

== matlab function double_pend/inv model 1/M1 ==
  data: m input; l input; q input; y output
function y = fcn(m, l, q)


y = [ (m(1)+m(2)) *l(1), m(2)*cos(q(1)-q(2)); m(2)*l(1)*cos(q(1)-q(2)), m(2)*l(2)] ;
